simulink model "motor_module"  (R2023b)
settings: Solver=ode4  StartTime=0.0  StopTime=0.5  FixedStep=0.0000002  RelTol=1e-3
libraries: spsFirstOrderFilterLib x2, simulink x2, spsDCVoltageSourceLib x1, spsGroundLib x1, spsPermanentMagnetSynchronousMachineLib x1, spsSVPWMGenerator2LevelLib x1, spsUniversalBridgeLib x1, spsdq0toAlphaBetaZeroLib x1, sps_lib x1
settings Model: Creator=user  LastModifiedBy=user

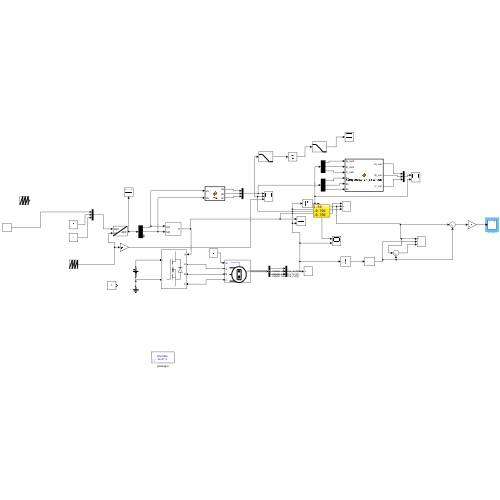
[thumbnail: Simulink's stored preview of the top-level diagram]
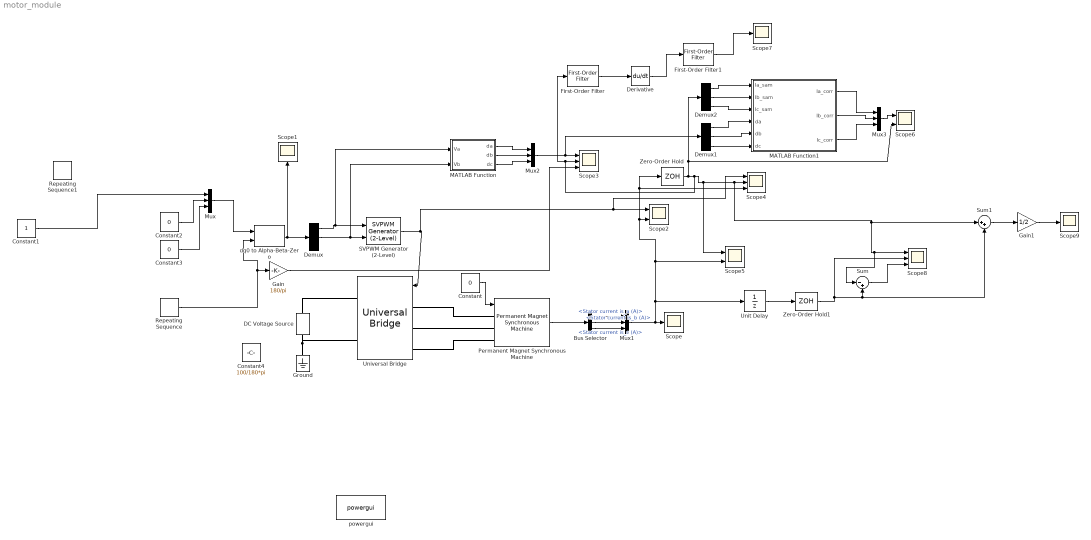
== system motor_module ==
  Bus Selector : BusSelector  OutputSignals=Stator current is_a (A),Stator current is_b (A),Stator current is_c (A)
  Constant : Constant  Value=0
  Constant1 : Constant
  Constant2 : Constant  Value=0
  Constant3 : Constant  Value=0
  Constant4 : Constant  Value=100/180*pi
  DC Voltage Source : spsDCVoltageSourceLib/DC Voltage Source  Amplitude=56  Measurements=None
  Demux : Demux  Outputs=3
  Demux1 : Demux  Outputs=3
  Demux2 : Demux  Outputs=3
  Derivative : Derivative
  First-Order Filter : spsFirstOrderFilterLib/First-Order Filter  FilterType=Lowpass  Tc=10e-4  Ts=0  Initialize=on  Vac_Init=[0, 0, 60]  Vdc_Init=0  PlotResponse=off  FreqRange="[0,  200,  1]"
  First-Order Filter1 : spsFirstOrderFilterLib/First-Order Filter  FilterType=Lowpass  Tc=10e-3  Ts=0  Initialize=on  Vac_Init=[0, 0, 60]  Vdc_Init=0  PlotResponse=off  FreqRange="[0,  200,  1]"
  Gain : Gain  Gain=180/pi
  Gain1 : Gain  Gain=1/2
  Ground : spsGroundLib/Ground  LConnTagsString=a
  MATLAB Function : MATLAB Function  TreatAsAtomicUnit=on
  MATLAB Function1 : MATLAB Function  TreatAsAtomicUnit=on
  Mux{,1..3} (4 alike) : Mux  Inputs=3
  Permanent Magnet Synchronous Machine : spsPermanentMagnetSynchronousMachineLib/Permanent Magnet Synchronous Machine  NbPhases=3  FluxDistribution=Sinusoidal  RotorType=Round  MechanicalLoad=Speed w  PresetModel=No  ShowDetailedParameters=on  MeasurementBus=off  Resistance=20  Inductance=8.5e-3  dqInductances=[8.5e-3,8.5e-3]  La=0.0006  MachineConstant=Flux linkage established by magnets (V.s)  Flux=0.1194  VoltageCst=86.6271  TorqueCst=0.7164  Flat=120  Mechanical=[0.0027 0.0004924 4 0]  PolePairs=4  InitialConditions=[0,0, 0,0]  InitialConditions5ph=[0 0 0 0 0 0]  RefAngle=Aligned with phase A axis (original Park)  IterativeDiscreteModel=Trapezoidal non iterative  TsBlock=-1  TsPowergui=0
  Repeating Sequence : simulink/Sources/Repeating Sequence  rep_seq_t=[0 0.5]  rep_seq_y=[0 2*pi]
  Repeating Sequence1 : simulink/Sources/Repeating Sequence  rep_seq_t=[0 0.5]  rep_seq_y=[0 1]
  SVPWM Generator (2-Level) : spsSVPWMGenerator2LevelLib/SVPWM Generator (2-Level)  InputType=alpha-beta components  SwitchingPattern=Pattern #1  Fc=10000  ParUref=[0.8 -30 50]  Ts=0
  Scope{,1,7,9} (4 alike) : Scope
  Scope2 : Scope  NumInputPorts=2
  Scope3 : Scope  NumInputPorts=3
  Scope4 : Scope  NumInputPorts=3
  Scope5 : Scope  NumInputPorts=2
  Scope6 : Scope  NumInputPorts=2
  Scope8 : Scope  NumInputPorts=3
  Sum : Sum  Inputs=|-+
  Sum1 : Sum  Inputs=|++
  Unit Delay : UnitDelay  SampleTime=0.00005  HasFrameUpgradeWarning=on
  Universal Bridge : spsUniversalBridgeLib/Universal Bridge  Arms=3  SnubberResistance=1e5  SnubberCapacitance=inf  Device=MOSFET / Diodes  Ron=1e-3  Lon=0  ForwardVoltages="[  0  0  ]"  ForwardVoltage=0  GTOparameters=[ 10e-6 , 20e-6 ]  IGBTparameters=[ 1e-6 , 2e-6 ]  Measurements=None  Measurements_2=None  converterType=Rectifier
  Zero-Order Hold : ZeroOrderHold  SampleTime=0.0001
  Zero-Order Hold1 : ZeroOrderHold  SampleTime=0.0001
  dq0 to Alpha-Beta-Zero : spsdq0toAlphaBetaZeroLib/dq0 to Alpha-Beta-Zero  Alignment=Aligned with phase A axis
  powergui : sps_lib/powergui  Priority=1  SimulationMode=Discrete  SampleTime=0.0000002  frequency=60  Iterations=50  frequencyindice=0  Pbase=100e6  ErrMax=1e-4  UnitsV=kV  UnitsW=MW  buscounter=0  FunctionMessages=off  echomessages=off  EnableUseOfTLC=off  CurrentSourceSwitches=off  DisableSnubberDevices=off  DisableRonSwitches=off  DisableVfSwitches=off  DisplayEquations=off  AutomaticDiscreteSolvers=off  SolverType=Tustin/Backward Euler (TBE)  Interpol=off  ExternalGateDelay=off  methode=off  Ts=100  x0status=blocks  SPID=on  SwTol=0  HookPort=off  NonlinearTolerance=1e-4  nMaxIteration=100  ContinueOnMaxIteration=off  RestoreLinks=warning  ResistiveCurrentMeasurement=off  Frange=[0:2:500]  Ylog=off  Xlog=on  ShowGrid=off  save=off  variable=ZData  structure=0  ZoomFFT=off  StartTime=0.0  cycles=1  DisplayStyle=1  fundamental=60  FreqAxis=off  MaxFrequency=1000  frequencyindicesteady=1  RmsSteady=1  display=off
  wires:
  Constant/1 -> Permanent Magnet Synchronous Machine/1
  dq0 to Alpha-Beta-Zero/1 -> Demux/1, Scope1/1
  Demux/1 -> MATLAB Function/1(Va), SVPWM Generator (2-Level)/1
  Demux/2 -> MATLAB Function/2(Vb), SVPWM Generator (2-Level)/2
  Constant2/1 -> Mux/2
  Mux/1 -> dq0 to Alpha-Beta-Zero/1
  Constant3/1 -> Mux/3
  SVPWM Generator (2-Level)/1 -> Scope4/1, Scope2/1, Universal Bridge/1
  Permanent Magnet Synchronous Machine/1 -> Bus Selector/1
  Mux1/1 -> Unit Delay/1, Scope5/2, Scope4/3, Zero-Order Hold/1, Scope2/2, Scope/1
  Bus Selector/2 -> Mux1/2  "<Stator current is_b (A)>"
  Bus Selector/1 -> Mux1/1  "<Stator current is_a (A)>"
  Bus Selector/3 -> Mux1/3  "<Stator current is_c (A)>"
  Mux2/1 -> Demux1/1, Scope3/1
  MATLAB Function/3(dc) -> Mux2/3
  MATLAB Function/2(db) -> Mux2/2
  MATLAB Function/1(da) -> Mux2/1
  Zero-Order Hold/1 -> Demux2/1, Scope6/2, First-Order Filter/1, Scope3/2, Scope5/1, Sum/1, Scope8/1, Sum1/1, Scope4/2
  Demux1/1 -> MATLAB Function1/4(da)
  Demux1/2 -> MATLAB Function1/5(db)
  Demux1/3 -> MATLAB Function1/6(dc)
  Demux2/1 -> MATLAB Function1/1(Ia_sam)
  Demux2/2 -> MATLAB Function1/2(Ib_sam)
  Demux2/3 -> MATLAB Function1/3(Ic_sam)
  MATLAB Function1/1(Ia_corr) -> Mux3/1
  MATLAB Function1/2(Ib_corr) -> Mux3/2
  MATLAB Function1/3(Ic_corr) -> Mux3/3
  Mux3/1 -> Scope6/1
  Gain/1 -> Scope3/3
  First-Order Filter/1 -> Derivative/1
  First-Order Filter1/1 -> Scope7/1
  Derivative/1 -> First-Order Filter1/1
  Unit Delay/1 -> Zero-Order Hold1/1
  Zero-Order Hold1/1 -> Sum1/2, Sum/2, Scope8/2
  Sum/1 -> Scope8/3
  Repeating Sequence/1 -> dq0 to Alpha-Beta-Zero/2, Gain/1
  Sum1/1 -> Gain1/1
  Gain1/1 -> Scope9/1
  Constant1/1 -> Mux/1
  connections:
  Universal Bridge/LConn1 -- Permanent Magnet Synchronous Machine/LConn1
  Universal Bridge/LConn2 -- Permanent Magnet Synchronous Machine/LConn2
  Universal Bridge/LConn3 -- Permanent Magnet Synchronous Machine/LConn3
  DC Voltage Source/LConn1 -- Universal Bridge/RConn2 -- Ground/LConn1
  Universal Bridge/RConn1 -- DC Voltage Source/RConn1

== matlab function motor_module/MATLAB Function1 ==
  data: Ia_sam input; Ia_corr output; Ib_sam input; Ib_corr output; Ic_corr output; Ic_sam input; da input; db input; dc input
function [Ia_corr, Ib_corr, Ic_corr] = compensate_LR_distortion(Ia_sam, Ib_sam, Ic_sam, da, db, dc)
    % COMPENSATE_LR_DISTORTION 修正由于 L/R 时间常数导致的采样电流畸变
    % 输入参数:
    %   I_sam: 低电平中心点采样的原始电流 (A)
    %   d: 0.0 ~ 1.0 的实时占空比指令
    
    %% 1. 系统参数标定 (根据实际硬件调整)
    % Vdc = 56V, Fsw = 10kHz, L = 0.6mH
    Vdc = 56;
    Fsw = 10000;
    L = 0.0006;
    Tsw = 1/Fsw;
    
    % K_BASE: 理想状态下的半纹波补偿系数 (Vdc*Tsw)/(2L)
    k_base = (Vdc * Tsw) / (2 * L);
    
    % K_LR: 针对 R 压降和指数衰减引入的二次/三次修正系数 (需标定)
    % 用于解决 Vq=0.95 时的波峰内凹畸变
    k_lr = 0.15; 
    
    %% 2. 核心物理补偿计算
    % 使用 D-0.5 描述占空比相对于对称点的偏离程度
    d_off_a = da - 0.5;
    d_off_b = db - 0.5;
    d_off_c = dc - 0.5;

    % 纹波包络项: D*(1-D) 决定了基础纹波厚度
    ripple_a = da * (1 - da);
    ripple_b = db * (1 - db);
    ripple_c = dc * (1 - dc);

    % 3. 构造补偿因子 (联合函数)
    % 结合了线性纹波项和针对 L/R 畸变的三次项拟合
    comp_a = k_base * ripple_a + k_lr * (d_off_a^3);
    comp_b = k_base * ripple_b + k_lr * (d_off_b^3);
    comp_c = k_base * ripple_c + k_lr * (d_off_c^3);

    %% 4. 对称性与过零点处理 (物理还原)
    % I_limit 定义过零平滑区，解决 image_4e6cad 中的台阶阶跃问题
    I_limit = 0.2; 
    
    % 正电流向上补，负电流向下补，恢复上下波形一致性
    % 使用 tanh 实现过零点的“软着陆”，确保修正前后波形在零点重叠
    Ia_corr = Ia_sam + tanh(Ia_sam / I_limit) * comp_a;
    Ib_corr = Ib_sam + tanh(Ib_sam / I_limit) * comp_b;
    Ic_corr = Ic_sam + tanh(Ic_sam / I_limit) * comp_c;
    
end

== matlab function motor_module/MATLAB Function ==
  data: Va input; da output; Vb input; db output; dc output
function [da, db, dc] = fcn(Va, Vb)
    % 输入: Va, Vb 范围为 -1 ~ 1
    
    % 1. Inverse Clarke 变换
    Vas = Va;
    Vbs = -0.5*Va + 0.8660254*Vb;
    Vcs = -0.5*Va - 0.8660254*Vb;
    
    % 2. SVPWM 零序注入 (注入 Min-Max 的均值)
    % 这一步能保证在不增加母线电压的情况下，获得最大的线性输出范围
    Vmax = max([Vas, Vbs, Vcs]);
    Vmin = min([Vas, Vbs, Vcs]);
    Vzero = 0.5 * (Vmax + Vmin);
    
    % 3. 生成马鞍波调制信号 (范围仍为 -1 ~ 1)
    Ta_saddle = Vas - Vzero;
    Tb_saddle = Vbs - Vzero;
    Tc_saddle = Vcs - Vzero;
    
    % 4. 归一化映射：将 [-1, 1] 映射到 [0, 1]
    % 公式：Duty = (Mod + 1) / 2
    da = (Ta_saddle + 1) / 2;
    db = (Tb_saddle + 1) / 2;
    dc = (Tc_saddle + 1) / 2;
    
    % 5. 严格限幅保护 (防止浮点数计算微量溢出)
    da = max(0, min(1, da));
    db = max(0, min(1, db));
    dc = max(0, min(1, dc));
end
